simulink model "Flap"  (R2024b)
settings: Solver=ode45  StartTime=0  StopTime=400  FixedStep=0.1  MaxStep=0.1  EnableMultiTasking=on
values from neighbouring files (symbols this model uses):
  Ki = -2*pi/5*imag(1/H(1)')    [BranchAndBound.m]    (also in Optimization.m; RectangularOptimization.m; RoundingPI.m; wecSimInputFile.m = -100000)
  Kp = real(1/H(1)')    [BranchAndBound.m]    (also in Optimization.m; RectangularOptimization.m; RoundingPI.m; wecSimInputFile.m = 500000)
  params = struct    [BranchAndBound.m]    (also in Optimization.m; Parameters.m = struct(); RectangularOptimization.m; RoundingPI.m)
  PTO = 'Continuous PI'    [wecSimInputFile.m]
  valveTransferFunction = tf(4/valveSettlingTime,[1 4/valveSettlingTime])    [Parameters.m]
undefined symbols (not defined in the file or in its folder): body, constraint, geometry, hydroData, pressure, pto, ptoSim
libraries: WECSim_Lib_Body_Elements x2, WECSim_Lib_Constraints x1, WECSim_Lib_Frames x1, simulink x1, WECSim_Lib_PTOSim x1, WECSim_Lib_PTOs x1
(part 1 of 2)
settings Model: Creator=mlawson  LastModifiedBy=jackson
settings SolverCC: ZeroCrossControl=DisableAll  AlgebraicLoopSolver=LineSearch  AutoInsertRateTranBlk=on
settings DataIOCC: SaveFormat=Array  SaveOutput=off  SaveTime=off  ReturnWorkspaceOutputs=off
settings OptimizationCC: LifeSpan=inf  SimCompilerOptimization=on
settings DebuggingCC: MergeDetectMultiDrivingBlocksExec=none  SolverPrmCheckMsg=warning  UnconnectedInputMsg=warning  UnconnectedOutputMsg=warning  UnconnectedLineMsg=warning  AllowSymbolicDim=off  StateNameClashWarn=warning  SFUnexpectedBacktrackingDiag=warning  SFNoUnconditionalDefaultTransitionDiag=warning  SFExecutionAtInitializationDiag=none  ArithmeticOperatorsInVariantConditions=warning
settings HardwareCC: ProdBitPerPointer=32  ProdBitPerSizeT=32  ProdBitPerPtrDiffT=32  ProdLargestAtomicFloat=None  ProdIntDivRoundTo=Undefined  ProdEndianess=Unspecified  ProdWordSize=32  ProdHWDeviceType=32-bit Generic
settings ModelReferenceCC: EnableRefExpFcnMdlSchedulingChecks=on  PropagateSignalLabelsOutOfModel=off
settings SFSimCC: SimUseLocalCustomCode=off  CustomCodeUndefinedFunction=UseInterfaceOnly
settings RTWCC: RTWUseLocalCustomCode=off  GPUComputeCapability=3.5  DLArmComputeVersion=19.05
settings CodeAppCC: StateflowObjectComments=on
settings GRTTargetCC: TargetLangStandard=C89/C90 (ANSI)
settings ConfigComp: CovMetricSettings=dw  CovSaveCumulativeToWorkspaceVar=on  CovSaveSingleToWorkspaceVar=on  CovExternalEMLEnable=off  CovSFcnEnable=off
settings SimscapeCC: SimscapeNormalizeSystem=off
settings ConfigurationSet: Description=SimMechanics 2G
settings ExplorerConfigSet: InternalSimMechanicsExplorerSettings="<ExplorerConfiguration><canonicalview>default</canonicalview><TilePanel><TileInfo><Tiles Columns=\"1\" Count=\"1\" Rows=\"1\"><Column Left=\"2\" Weight=\"1\"/><Column Left=\"1335\"/><Row Top=\"2\" Weight=\"1\"/><Row Top=\"911\"/><Tile Height=\"1\" Width=\"1\" X=\"0\" Y=\"0\"/></Tiles></TileInfo><SceneInfo><SceneViewer><BGColor><R>0.60000002384185791</R><G>0.60000002384185791</G><B>0.60000002384185791</B></BGColor><Camera><Position><X>365.37645888990272</X><Y>-369.82486814446582</Y><Z>359.64809521743916</Z></Position><Center><X>-6.7351450971904585</X><Y>2.2867358426280204</Y><Z>-12.463508769654169</Z></Center><Up><X>-0.40824829046386307</X><Y>0.40824829046386307</Y><Z>0.81649658092772615</Z></Up><Left>-57.820127362122818</Left><Right>57.820127362122818</Right><Bottom>-38.308817187253304</Bottom><Top>38.308817187253304</Top></Camera></SceneViewer></SceneInfo></TilePanel></ExplorerConfiguration>"

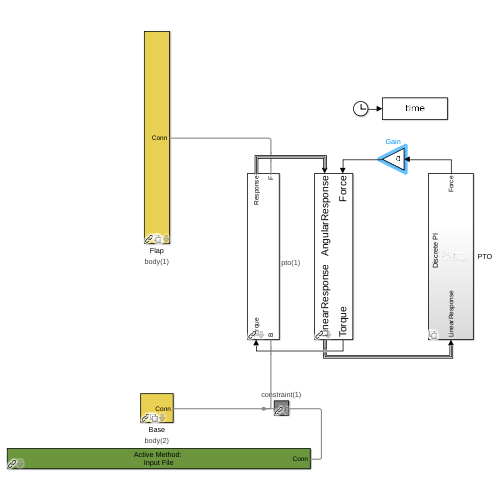
[thumbnail: Simulink's stored preview of the top-level diagram]
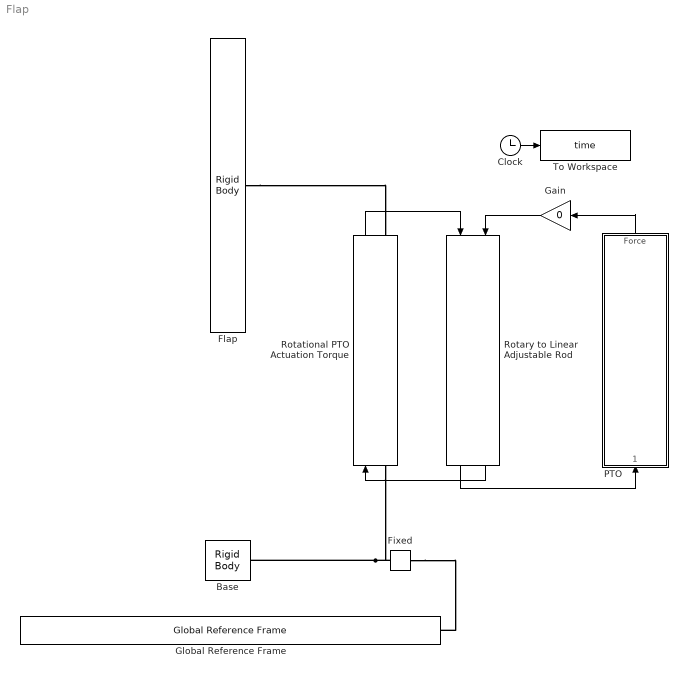
== system Flap ==
  Base : WECSim_Lib_Body_Elements/Rigid Body  body=body(2)  h5File=hydroData/*.h5  geometryFile=geometry/*.stl  mass=0  inertia=0 0 0  inertiaProducts=0 0 0  nonHydro=0  nonlinearHydro=0  centerGravity=0 0 0  centerBuoyancy=0 0 0  dof=6  volume=0  QTFs=0  displacement=0 0 0  axis=0 1 0  angle=0  option=0  cd=0 0 0  ca=0 0 0  area=0 0 0  VME=0  rgME=0 0 0  z=0 0 1
      settings: SourceProductName=WEC-Sim
  Clock : Clock
  Fixed : WECSim_Lib_Constraints/Fixed  constraint=constraint(1)  loc="0  0  0"  displacement=0 0 0  y=0 1 0  z=0 0 1  upperLimitSpecify=off  upperLimitBound=0  upperLimitTransitionRegionWidth=0  upperLimitStiffness=0  upperLimitDamping=0  lowerLimitSpecify=off  lowerLimitBound=0  lowerLimitTransitionRegionWidth=0  lowerLimitStiffness=0  lowerLimitDamping=0
      settings: AttributesFormatString=%<constraint>  SourceProductName=WEC-Sim
  Flap : WECSim_Lib_Body_Elements/Rigid Body  body=body(1)  h5File=hydroData/*.h5  geometryFile=geometry/*.stl  mass=0  inertia=0 0 0  inertiaProducts=0 0 0  nonHydro=0  nonlinearHydro=0  centerGravity=0 0 0  centerBuoyancy=0 0 0  dof=6  volume=0  QTFs=0  displacement=0 0 0  axis=0 1 0  angle=0  option=0  cd=0 0 0  ca=0 0 0  area=0 0 0  VME=0  rgME=0 0 0  z=0 0 1
      settings: SourceProductName=WEC-Sim
  Gain : Gain  Gain=0
  Global Reference Frame : WECSim_Lib_Frames/Global Reference Frame  waves=waves  simu=simu  InputMethod=Input File  InputFile=wecSimInputFile.m  mode=normal  explorer=off  solver=ode4  startTime=0  rampTime=100  endTime=400  dt=0.1  cicEndTime=60  stateSpace=0  WaveClass=regular  height=2.5  period=8  elevationFile=NOT DEFINED  spectrumFile=NOT DEFINED  direction=0  spread=1  spectrumType=NOT DEFINED  phaseSeed=0  option=EqualEnergy
      settings: SourceProductName=WEC-Sim
  PTO : Subsystem  Variant=on
  Rotary to Linear Adjustable Rod : WECSim_Lib_PTOSim/Motion Conversion/Rotary to Linear Adjustable Rod  ptoSim=ptoSim(1)  crank=crank_z  offset=0  rodInit=initalCylinderLength
  Rotational PTO Actuation Torque : WECSim_Lib_PTOs/Rotational PTO Actuation Torque  pto=pto(1)  loc="0  0  0"  stiffness=0  damping=0  equilibriumPosition=0  pretension=0  displacement=0 0 0  y=0 1 0  z=0 0 1  upperLimitSpecify=off  upperLimitBound=0  upperLimitTransitionRegionWidth=0  upperLimitStiffness=0  upperLimitDamping=0  lowerLimitSpecify=off  lowerLimitBound=0  lowerLimitTransitionRegionWidth=0  lowerLimitStiffness=0  lowerLimitDamping=0
      settings: AttributesFormatString=%<pto>
  To Workspace : ToWorkspace  VariableName=time  SampleTime=-1
  wires:
  Rotational PTO Actuation Torque/1 -> Rotary to Linear Adjustable Rod/1
  Rotary to Linear Adjustable Rod/2 -> Rotational PTO Actuation Torque/1
  Rotary to Linear Adjustable Rod/1 -> PTO/1(LinearResponse)
  PTO/1(Force) -> Gain/1
  Clock/1 -> To Workspace/1
  Gain/1 -> Rotary to Linear Adjustable Rod/2
  connections:
  Fixed/LConn1 -- Global Reference Frame/RConn1
  Fixed/RConn1 -- Base/RConn1 -- Rotational PTO Actuation Torque/LConn1
  Flap/RConn1 -- Rotational PTO Actuation Torque/RConn1

== system Flap/PTO ==
  note: 1) Add Subsystem or Model blocks as valid variant choices.
      | 2) You cannot connect blocks at this level. At simulation, connectivity is automatically
      | determined, based on the active variant and port name matching.
  LinearResponse : Inport
  Active Valving : Subsystem  VariantControl=strcmp(PTO, 'Active Valving')
  Continuous PI : Subsystem  VariantControl=strcmp(PTO, 'Continuous PI')
  Discrete PI : Subsystem  VariantControl=strcmp(PTO, 'Discrete PI')
  EHA : Subsystem  VariantControl=strcmp(PTO, 'EHA')
  HHEA : Subsystem  VariantControl=strcmp(PTO, 'HHEA')
  Passive Valving : Subsystem  VariantControl=strcmp(PTO, 'Passive Valving')
  Rectifying : Subsystem  VariantControl=strcmp(PTO, 'Rectifying')
  Force : Outport

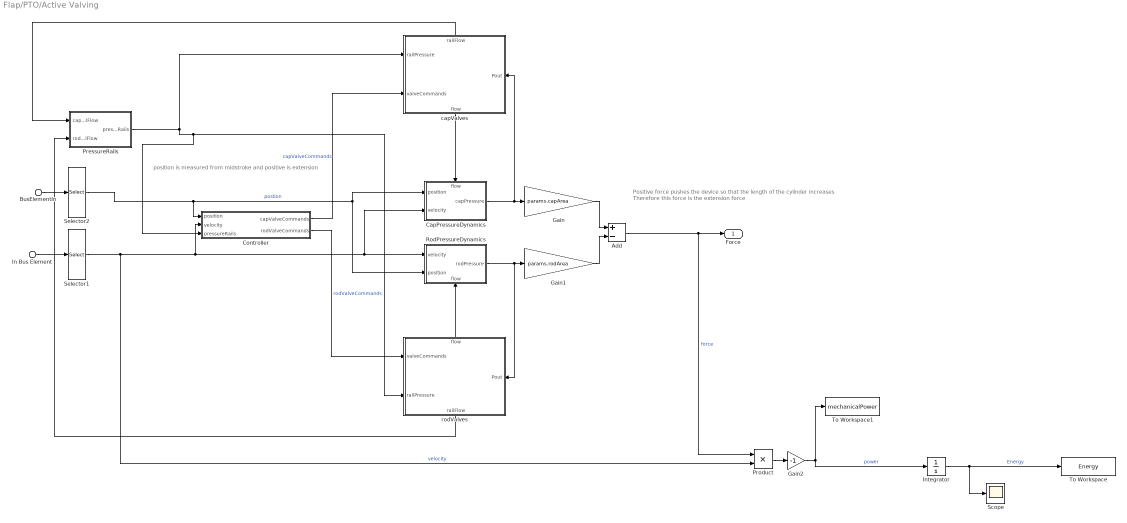
== system Flap/PTO/Active Valving ==
  note: position is measured from midstroke and positive is extension
  note: Positive force pushes the device so that the length of the cylinder increases
      | Therefore this force is the extension force
  In Bus Element : Inport  PortName=LinearResponse  Element=velocity
  BusElementIn : Inport  PortName=LinearResponse  Element=position
  Add : Sum  Inputs=+-
  CapPressureDynamics : Subsystem
      settings: PortSchema="{\"entries\":[{\"content\":{\"sides\":[{\"content\":{\"connectorIds\":[\"In1\",\"In2\"]},\"type\":\"ConnectorPlacement.EquallySpacedRectSide\",\"uuid\":\"0a444e4d-7364-44e5-8b72-8c210fabafa0\"},{\"content\":{\"connectorIds\":[\"Out1\"],\"side\":\"RIGHT\"},\"type\":\"ConnectorPlacement.EquallySpacedRectSide\",\"uuid\":\"a3669697-8e2e-4fce-83e7-11feb3c41a11\"},{\"content\":{\"connectorIds\":[\"In3\"],\"side\":\"TOP\"},\"type\":\"ConnectorPlacement.EquallySpacedRectSide\",\"uuid\":\"edbd7469-179d-4b36-ab80-dceaa86ef763\"},{\"content\":{\"side\":\"BOTTOM\"},\"type\":\"ConnectorPlacement.EquallySpacedRectSide\",\"uuid\":\"36ba3990-6628-4e3d-ab1a-10917dd4fa0b\"}]},\"type\":\"ConnectorPlacement.EquallySpacedConnector\",\"uuid\":\"68480e3c-12c2-4c1a-9580-60c15ea9a162\"}],\"packageUris\":[\"http://schema.mathworks.com/mf0/Connector/R2020b\"],\"version\":\"1.0\"}"
  Controller : Subsystem
  Gain : Gain  Gain=params.capArea
  Gain1 : Gain  Gain=params.rodArea
  Gain2 : Gain  Gain=-1
  Integrator : Integrator
  PressureRails : Subsystem
  Product : Product
  RodPressureDynamics : Subsystem
      settings: PortSchema="{\"entries\":[{\"content\":{\"sides\":[{\"content\":{\"connectorIds\":[\"In1\",\"In2\"]},\"type\":\"ConnectorPlacement.EquallySpacedRectSide\",\"uuid\":\"0a444e4d-7364-44e5-8b72-8c210fabafa0\"},{\"content\":{\"connectorIds\":[\"Out1\"],\"side\":\"RIGHT\"},\"type\":\"ConnectorPlacement.EquallySpacedRectSide\",\"uuid\":\"a3669697-8e2e-4fce-83e7-11feb3c41a11\"},{\"content\":{\"side\":\"TOP\"},\"type\":\"ConnectorPlacement.EquallySpacedRectSide\",\"uuid\":\"edbd7469-179d-4b36-ab80-dceaa86ef763\"},{\"content\":{\"connectorIds\":[\"In3\"],\"side\":\"BOTTOM\"},\"type\":\"ConnectorPlacement.EquallySpacedRectSide\",\"uuid\":\"0057cc85-602f-4ff7-8e06-c43254199496\"}]},\"type\":\"ConnectorPlacement.EquallySpacedConnector\",\"uuid\":\"68480e3c-12c2-4c1a-9580-60c15ea9a162\"}],\"packageUris\":[\"http://schema.mathworks.com/mf0/Connector/R2020b\"],\"version\":\"1.0\"}"
  Scope : Scope
  Selector1 : Selector  InputPortWidth=6  IndexOptions=Index vector (dialog)  Indices=3  OutputSizes=1
  Selector2 : Selector  InputPortWidth=6  IndexOptions=Index vector (dialog)  Indices=3  OutputSizes=1
  To Workspace : ToWorkspace  VariableName=Energy  SampleTime=-1
      settings: MaxDataPoints=1
  To Workspace1 : ToWorkspace  VariableName=mechanicalPower  SampleTime=-1
  capValves : Subsystem
      settings: PortSchema="{\"entries\":[{\"content\":{\"sides\":[{\"content\":{\"connectorIds\":[\"In1\",\"In2\"]},\"type\":\"ConnectorPlacement.EquallySpacedRectSide\",\"uuid\":\"d2e8cfa0-a0ae-49da-8fda-082dfd3b2d9f\"},{\"content\":{\"connectorIds\":[\"In3\"],\"side\":\"RIGHT\"},\"type\":\"ConnectorPlacement.EquallySpacedRectSide\",\"uuid\":\"7b83af61-76d6-4e35-9365-fafdba130762\"},{\"content\":{\"connectorIds\":[\"Out2\"],\"side\":\"TOP\"},\"type\":\"ConnectorPlacement.EquallySpacedRectSide\",\"uuid\":\"6880d985-ed9d-415d-a1a9-fc8aaf1ae9e0\"},{\"content\":{\"connectorIds\":[\"Out1\"],\"side\":\"BOTTOM\"},\"type\":\"ConnectorPlacement.EquallySpacedRectSide\",\"uuid\":\"f70b92c7-c6bf-4dbf-a331-364ba55ce8fb\"}]},\"type\":\"ConnectorPlacement.EquallySpacedConnector\",\"uuid\":\"7ffcaf2b-fb7f-4cb0-b739-43ebea45fc90\"}],\"packageUris\":[\"http://schema.mathworks.com/mf0/Connector/R2020b\"],\"version\":\"1.0\"}"
  rodValves : Subsystem
      settings: PortSchema="{\"entries\":[{\"content\":{\"sides\":[{\"content\":{\"connectorIds\":[\"In1\",\"In2\"]},\"type\":\"ConnectorPlacement.EquallySpacedRectSide\",\"uuid\":\"d2e8cfa0-a0ae-49da-8fda-082dfd3b2d9f\"},{\"content\":{\"connectorIds\":[\"In3\"],\"side\":\"RIGHT\"},\"type\":\"ConnectorPlacement.EquallySpacedRectSide\",\"uuid\":\"7b83af61-76d6-4e35-9365-fafdba130762\"},{\"content\":{\"connectorIds\":[\"Out2\"],\"side\":\"TOP\"},\"type\":\"ConnectorPlacement.EquallySpacedRectSide\",\"uuid\":\"6880d985-ed9d-415d-a1a9-fc8aaf1ae9e0\"},{\"content\":{\"connectorIds\":[\"Out1\"],\"side\":\"BOTTOM\"},\"type\":\"ConnectorPlacement.EquallySpacedRectSide\",\"uuid\":\"f70b92c7-c6bf-4dbf-a331-364ba55ce8fb\"}]},\"type\":\"ConnectorPlacement.EquallySpacedConnector\",\"uuid\":\"7ffcaf2b-fb7f-4cb0-b739-43ebea45fc90\"}],\"packageUris\":[\"http://schema.mathworks.com/mf0/Connector/R2020b\"],\"version\":\"1.0\"}"
  Force : Outport
  wires:
  rodValves/2(flow) -> RodPressureDynamics/3(flow)
  Controller/2(rodValveCommands) -> rodValves/1(valveCommands)  "rodValveCommands"
  Controller/1(capValveCommands) -> capValves/2(valveCommands)  "capValveCommands"
  capValves/1(flow) -> CapPressureDynamics/3(flow)
  RodPressureDynamics/1(rodPressure) -> rodValves/3(Pout), Gain1/1
  PressureRails/1(pressureRails) -> capValves/1(railPressure), Controller/3(pressureRails), rodValves/2(railPressure)
  Gain1/1 -> Add/2
  CapPressureDynamics/1(capPressure) -> capValves/3(Pout), Gain/1
  Gain/1 -> Add/1
  BusElementIn/1 -> Selector2/1
  In Bus Element/1 -> Selector1/1
  Selector2/1 -> Controller/1(position), RodPressureDynamics/2(position), CapPressureDynamics/1(position)  "postion"
  Selector1/1 -> Product/2, Controller/2(velocity), RodPressureDynamics/1(velocity), CapPressureDynamics/2(velocity)  "velocity"
  Integrator/1 -> To Workspace/1, Scope/1  "Energy"
  Add/1 -> Product/1, Force/1  "force"
  rodValves/1(railFlow) -> PressureRails/2(rodRailFlow)
  capValves/2(railFlow) -> PressureRails/1(capRailFlow)
  Gain2/1 -> Integrator/1, To Workspace1/1  "power"
  Product/1 -> Gain2/1

== system Flap/PTO/Continuous PI ==
  note: Positive force pushes the device so that the length of the cylinder increases
      | Therefore this force is the extension force
  In Bus Element : Inport  PortName=LinearResponse  Element=velocity
  BusElementIn : Inport  PortName=LinearResponse  Element=position
  Gain : Gain  Gain=-Ki
  Gain1 : Gain  Gain=-Kp
  Integrator : Integrator
  Product : Product
  Scope : Scope
  Scope1 : Scope  NumInputPorts=2
  Selector1 : Selector  InputPortWidth=6  IndexOptions=Index vector (dialog)  Indices=3  OutputSizes=1
  Selector2 : Selector  InputPortWidth=6  IndexOptions=Index vector (dialog)  Indices=3  OutputSizes=1
  Sum : Sum  Inputs=|++
  To Workspace : ToWorkspace  VariableName=Energy  SampleTime=-1
      settings: MaxDataPoints=1
  Force : Outport
  wires:
  BusElementIn/1 -> Selector2/1
  In Bus Element/1 -> Selector1/1
  Sum/1 -> Scope1/1, Product/1, Force/1  "force"
  Selector1/1 -> Scope1/2, Gain1/1, Product/2  "velocity"
  Gain/1 -> Sum/1
  Gain1/1 -> Sum/2
  Product/1 -> Integrator/1  "Power"
  Integrator/1 -> To Workspace/1, Scope/1  "Energy"
  Selector2/1 -> Gain/1  "length"

== system Flap/PTO/Discrete PI ==
  note: Positive force pushes the device so that the length of the cylinder increases
      | Therefore this force is the extension force
  In Bus Element : Inport  PortName=LinearResponse  Element=velocity
  BusElementIn : Inport  PortName=LinearResponse  Element=position
  Gain : Gain  Gain=-Ki
  Gain1 : Gain  Gain=-Kp
  Integrator : Integrator
  MATLAB Function : MATLAB Function  TreatAsAtomicUnit=on
  Product : Product
  Scope : Scope
  Scope1 : Scope  NumInputPorts=2
  Selector1 : Selector  InputPortWidth=6  IndexOptions=Index vector (dialog)  Indices=3  OutputSizes=1
  Selector2 : Selector  InputPortWidth=6  IndexOptions=Index vector (dialog)  Indices=3  OutputSizes=1
  Sum : Sum  Inputs=|++
  To Workspace : ToWorkspace  VariableName=Energy  SampleTime=-1
      settings: MaxDataPoints=1
  Force : Outport
  wires:
  Integrator/1 -> To Workspace/1, Scope/1  "Energy"
  Product/1 -> Integrator/1  "Power"
  Gain1/1 -> Sum/2
  Gain/1 -> Sum/1
  Selector1/1 -> Gain1/1, Product/2  "velocity"
  Selector2/1 -> Gain/1  "length"
  Sum/1 -> Scope1/1, MATLAB Function/1(forceContinuous)  "ContinuousForce"
  In Bus Element/1 -> Selector1/1
  BusElementIn/1 -> Selector2/1
  MATLAB Function/1(forceDiscrete) -> Force/1, Scope1/2, Product/1  "discreteForce"

== system Flap/PTO/EHA ==
  In Bus Element : Inport  PortName=LinearResponse  Element=velocity
  BusElementIn : Inport  PortName=LinearResponse  Element=position
  Controller : Subsystem
  Selector1 : Selector  InputPortWidth=6  IndexOptions=Index vector (dialog)  Indices=3  OutputSizes=1
  Selector2 : Selector  InputPortWidth=6  IndexOptions=Index vector (dialog)  Indices=3  OutputSizes=1
  Subsystem : Subsystem
  Force : Outport
  wires:
  Subsystem/2(capPressure) -> Controller/3(capPressure)
  In Bus Element/1 -> Selector1/1  "velcty"
  Subsystem/1(Force) -> Force/1
  BusElementIn/1 -> Selector2/1
  Selector2/1 -> Controller/1(position), Subsystem/1(position)  "postion"
  Selector1/1 -> Subsystem/3(velocity), Controller/2(velocity)  "velocity"
  Controller/1(displacementCommand) -> Subsystem/2(displacementCommand)
  Subsystem/3(rodPressure) -> Controller/4(rodPressure)

== system Flap/PTO/HHEA ==
  In Bus Element : Inport  PortName=LinearResponse  Element=velocity
  BusElementIn : Inport  PortName=LinearResponse  Element=position
  Controller : Subsystem
  Selector1 : Selector  InputPortWidth=6  IndexOptions=Index vector (dialog)  Indices=3  OutputSizes=1
  Selector2 : Selector  InputPortWidth=6  IndexOptions=Index vector (dialog)  Indices=3  OutputSizes=1
  Subsystem : Subsystem
  Force : Outport
  wires:
  Controller/3("dP_command ") -> Subsystem/4("rodPressureCommand ")
  Subsystem/3(capPressure) -> Controller/4(capPressure)
  Controller/1(capValveCommands) -> Subsystem/2(capValveCommands)  "capValveCommands"
  Subsystem/4(rodValvePressure) -> Controller/5(rodValvePressure)
  In Bus Element/1 -> Selector1/1  "velcty"
  Subsystem/1(Force) -> Force/1
  Controller/2(rodValveCommands) -> Subsystem/3(rodValveCommands)  "rodValveCommands"
  BusElementIn/1 -> Selector2/1
  Subsystem/2(railPressure) -> Controller/3(pressureRails)
  Selector2/1 -> Controller/1(position), Subsystem/1(position)  "postion"
  Selector1/1 -> Subsystem/6(velocity), Controller/2(velocity)  "velocity"
  Controller/4(speedCommand) -> Subsystem/5(speedCommand)
  Subsystem/5(rodPressure) -> Controller/6(rodPressure)

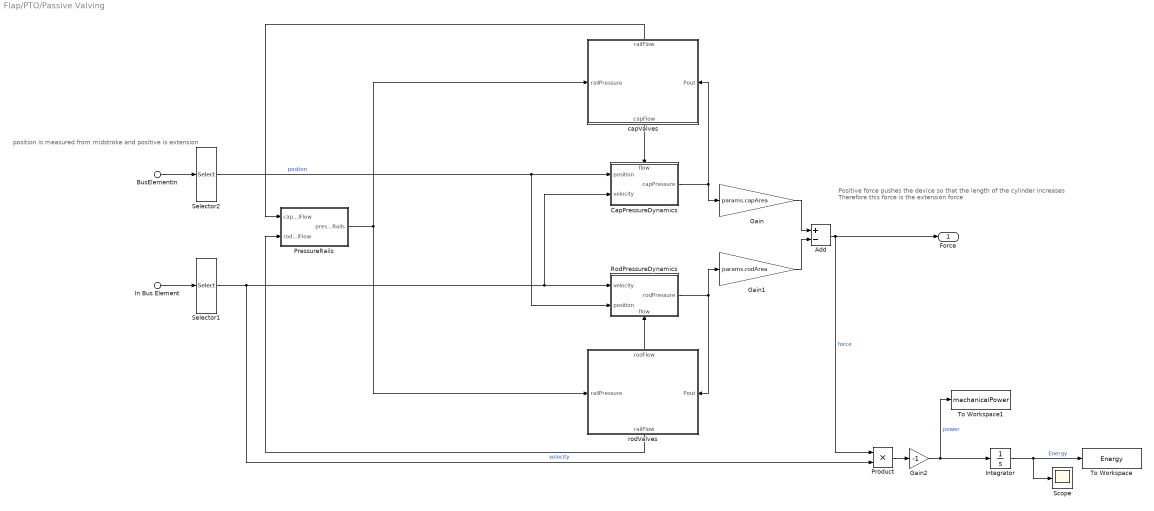
== system Flap/PTO/Passive Valving ==
  note: Positive force pushes the device so that the length of the cylinder increases
      | Therefore this force is the extension force
  note: position is measured from midstroke and positive is extension
  In Bus Element : Inport  PortName=LinearResponse  Element=velocity
  BusElementIn : Inport  PortName=LinearResponse  Element=position
  Add : Sum  Inputs=+-
  CapPressureDynamics : Subsystem
      settings: PortSchema="{\"entries\":[{\"content\":{\"sides\":[{\"content\":{\"connectorIds\":[\"In1\",\"In2\"]},\"type\":\"ConnectorPlacement.EquallySpacedRectSide\",\"uuid\":\"0a444e4d-7364-44e5-8b72-8c210fabafa0\"},{\"content\":{\"connectorIds\":[\"Out1\"],\"side\":\"RIGHT\"},\"type\":\"ConnectorPlacement.EquallySpacedRectSide\",\"uuid\":\"a3669697-8e2e-4fce-83e7-11feb3c41a11\"},{\"content\":{\"connectorIds\":[\"In3\"],\"side\":\"TOP\"},\"type\":\"ConnectorPlacement.EquallySpacedRectSide\",\"uuid\":\"edbd7469-179d-4b36-ab80-dceaa86ef763\"},{\"content\":{\"side\":\"BOTTOM\"},\"type\":\"ConnectorPlacement.EquallySpacedRectSide\",\"uuid\":\"36ba3990-6628-4e3d-ab1a-10917dd4fa0b\"}]},\"type\":\"ConnectorPlacement.EquallySpacedConnector\",\"uuid\":\"68480e3c-12c2-4c1a-9580-60c15ea9a162\"}],\"packageUris\":[\"http://schema.mathworks.com/mf0/Connector/R2020b\"],\"version\":\"1.0\"}"
  Gain : Gain  Gain=params.capArea
  Gain1 : Gain  Gain=params.rodArea
  Gain2 : Gain  Gain=-1
  Integrator : Integrator
  PressureRails : Subsystem
  Product : Product
  RodPressureDynamics : Subsystem
      settings: PortSchema="{\"entries\":[{\"content\":{\"sides\":[{\"content\":{\"connectorIds\":[\"In1\",\"In2\"]},\"type\":\"ConnectorPlacement.EquallySpacedRectSide\",\"uuid\":\"0a444e4d-7364-44e5-8b72-8c210fabafa0\"},{\"content\":{\"connectorIds\":[\"Out1\"],\"side\":\"RIGHT\"},\"type\":\"ConnectorPlacement.EquallySpacedRectSide\",\"uuid\":\"a3669697-8e2e-4fce-83e7-11feb3c41a11\"},{\"content\":{\"side\":\"TOP\"},\"type\":\"ConnectorPlacement.EquallySpacedRectSide\",\"uuid\":\"edbd7469-179d-4b36-ab80-dceaa86ef763\"},{\"content\":{\"connectorIds\":[\"In3\"],\"side\":\"BOTTOM\"},\"type\":\"ConnectorPlacement.EquallySpacedRectSide\",\"uuid\":\"0057cc85-602f-4ff7-8e06-c43254199496\"}]},\"type\":\"ConnectorPlacement.EquallySpacedConnector\",\"uuid\":\"68480e3c-12c2-4c1a-9580-60c15ea9a162\"}],\"packageUris\":[\"http://schema.mathworks.com/mf0/Connector/R2020b\"],\"version\":\"1.0\"}"
  Scope : Scope
  Selector1 : Selector  InputPortWidth=6  IndexOptions=Index vector (dialog)  Indices=3  OutputSizes=1
  Selector2 : Selector  InputPortWidth=6  IndexOptions=Index vector (dialog)  Indices=3  OutputSizes=1
  To Workspace : ToWorkspace  VariableName=Energy  SampleTime=-1
      settings: MaxDataPoints=1
  To Workspace1 : ToWorkspace  VariableName=mechanicalPower  SampleTime=-1
  capValves : Subsystem
      settings: PortSchema="{\"entries\":[{\"content\":{\"sides\":[{\"content\":{\"connectorIds\":[\"In1\"]},\"type\":\"ConnectorPlacement.EquallySpacedRectSide\",\"uuid\":\"d2e8cfa0-a0ae-49da-8fda-082dfd3b2d9f\"},{\"content\":{\"connectorIds\":[\"In2\"],\"side\":\"RIGHT\"},\"type\":\"ConnectorPlacement.EquallySpacedRectSide\",\"uuid\":\"7b83af61-76d6-4e35-9365-fafdba130762\"},{\"content\":{\"connectorIds\":[\"Out2\"],\"side\":\"TOP\"},\"type\":\"ConnectorPlacement.EquallySpacedRectSide\",\"uuid\":\"6880d985-ed9d-415d-a1a9-fc8aaf1ae9e0\"},{\"content\":{\"connectorIds\":[\"Out1\"],\"side\":\"BOTTOM\"},\"type\":\"ConnectorPlacement.EquallySpacedRectSide\",\"uuid\":\"f70b92c7-c6bf-4dbf-a331-364ba55ce8fb\"}]},\"type\":\"ConnectorPlacement.EquallySpacedConnector\",\"uuid\":\"7ffcaf2b-fb7f-4cb0-b739-43ebea45fc90\"}],\"packageUris\":[\"http://schema.mathworks.com/mf0/Connector/R2020b\"],\"version\":\"1.0\"}"
  rodValves : Subsystem
      settings: PortSchema="{\"entries\":[{\"content\":{\"sides\":[{\"content\":{\"connectorIds\":[\"In1\"]},\"type\":\"ConnectorPlacement.EquallySpacedRectSide\",\"uuid\":\"d2e8cfa0-a0ae-49da-8fda-082dfd3b2d9f\"},{\"content\":{\"connectorIds\":[\"In2\"],\"side\":\"RIGHT\"},\"type\":\"ConnectorPlacement.EquallySpacedRectSide\",\"uuid\":\"7b83af61-76d6-4e35-9365-fafdba130762\"},{\"content\":{\"connectorIds\":[\"Out2\"],\"side\":\"TOP\"},\"type\":\"ConnectorPlacement.EquallySpacedRectSide\",\"uuid\":\"6880d985-ed9d-415d-a1a9-fc8aaf1ae9e0\"},{\"content\":{\"connectorIds\":[\"Out1\"],\"side\":\"BOTTOM\"},\"type\":\"ConnectorPlacement.EquallySpacedRectSide\",\"uuid\":\"f70b92c7-c6bf-4dbf-a331-364ba55ce8fb\"}]},\"type\":\"ConnectorPlacement.EquallySpacedConnector\",\"uuid\":\"7ffcaf2b-fb7f-4cb0-b739-43ebea45fc90\"}],\"packageUris\":[\"http://schema.mathworks.com/mf0/Connector/R2020b\"],\"version\":\"1.0\"}"
  Force : Outport
  wires:
  Add/1 -> Force/1, Product/1  "force"
  Product/1 -> Gain2/1
  Integrator/1 -> Scope/1, To Workspace/1  "Energy"
  Selector1/1 -> CapPressureDynamics/2(velocity), RodPressureDynamics/1(velocity), Product/2  "velocity"
  Selector2/1 -> RodPressureDynamics/2(position), CapPressureDynamics/1(position)  "postion"
  In Bus Element/1 -> Selector1/1
  BusElementIn/1 -> Selector2/1
  Gain/1 -> Add/1
  CapPressureDynamics/1(capPressure) -> Gain/1, capValves/2(Pout)
  Gain1/1 -> Add/2
  RodPressureDynamics/1(rodPressure) -> Gain1/1, rodValves/2(Pout)
  capValves/1(capFlow) -> CapPressureDynamics/3(flow)
  rodValves/2(rodFlow) -> RodPressureDynamics/3(flow)
  PressureRails/1(pressureRails) -> capValves/1(railPressure), rodValves/1(railPressure)
  capValves/2(railFlow) -> PressureRails/1(capRailFlow)
  rodValves/1(railFlow) -> PressureRails/2(rodRailFlow)
  Gain2/1 -> Integrator/1, To Workspace1/1  "power"

== system Flap/PTO/Rectifying ==
  note: Positive force pushes the device so that the length of the cylinder increases
      | Therefore this force is the extension force
  In Bus Element : Inport  PortName=LinearResponse  Element=velocity
  BusElementIn : Inport  PortName=LinearResponse  Element=position
  Constant : Constant  Value=pressure
  Integrator : Integrator
  MATLAB Function : MATLAB Function  TreatAsAtomicUnit=on
  Product : Product
  Scope : Scope
  Scope1 : Scope  NumInputPorts=2
  Selector1 : Selector  InputPortWidth=6  IndexOptions=Index vector (dialog)  Indices=3  OutputSizes=1
  Selector2 : Selector  InputPortWidth=6  IndexOptions=Index vector (dialog)  Indices=3  OutputSizes=1
  Terminator : Terminator
  To Workspace : ToWorkspace  VariableName=Energy  SampleTime=-1
      settings: MaxDataPoints=1
  Force : Outport
  wires:
  Integrator/1 -> To Workspace/1, Scope/1  "Energy"
  Product/1 -> Integrator/1  "Power"
  Selector1/1 -> MATLAB Function/1(velocity), Scope1/1, Product/2  "velocity"
  MATLAB Function/1(forceRectified) -> Scope1/2, Product/1, Force/1
  Constant/1 -> MATLAB Function/2(pressure)
  In Bus Element/1 -> Selector1/1
  BusElementIn/1 -> Selector2/1
  Selector2/1 -> Terminator/1  "position"

== system Flap/PTO/Active Valving/CapPressureDynamics ==
  position : Inport
  velocity : Inport  Port=2
  flow : Inport  Port=3
  Integrator : Integrator  LimitOutput=on  UpperSaturationLimit=40e6  LowerSaturationLimit=0
  MATLAB Function : MATLAB Function  TreatAsAtomicUnit=on
  capPressure : Outport
  wires:
  MATLAB Function/1(pressure_dot) -> Integrator/1
  Integrator/1 -> capPressure/1  "capPressure"
  flow/1 -> MATLAB Function/3(flow)
  velocity/1 -> MATLAB Function/2(velocity)
  position/1 -> MATLAB Function/1(position)

== system Flap/PTO/Active Valving/Controller ==
  position : Inport
  velocity : Inport  Port=2
  pressureRails : Inport  Port=3
  Gain : Gain  Gain=-params.Ki
  Gain1 : Gain  Gain=-params.Kp
  MATLAB Function : MATLAB Function  TreatAsAtomicUnit=on
  Scope1 : Scope  NumInputPorts=2
  Sum : Sum  Inputs=|++
  Terminator : Terminator
  Terminator1 : Terminator
  Zero-Order Hold : ZeroOrderHold  SampleTime=.2
  Zero-Order Hold1 : ZeroOrderHold  SampleTime=.2
  capValveCommands : Outport
  rodValveCommands : Outport  Port=2
  wires:
  velocity/1 -> Gain1/1  "velocity"
  Gain1/1 -> Sum/2
  Gain/1 -> Sum/1
  Sum/1 -> Scope1/1, MATLAB Function/1(forceContinuous)  "forceContinuous"
  MATLAB Function/3(forceDiscrete) -> Scope1/2  "forceDiscrete"
  position/1 -> Gain/1  "position"
  MATLAB Function/1(capValveCommands) -> Zero-Order Hold/1
  pressureRails/1 -> MATLAB Function/2(pressureRails)
  MATLAB Function/4(capPressureCommand) -> Terminator/1  "capPressureCommand"
  MATLAB Function/5(rodPressureCommand) -> Terminator1/1  "rodPressureCommand"
  Zero-Order Hold/1 -> capValveCommands/1
  MATLAB Function/2(rodValveCommands) -> Zero-Order Hold1/1
  Zero-Order Hold1/1 -> rodValveCommands/1

== system Flap/PTO/Active Valving/PressureRails ==
  note: flow into the rails
  capRailFlow : Inport
  rodRailFlow : Inport  Port=2
  Constant : Constant  Value=35e6
  Constant3 : Constant  Value=17.5e6
  Constant4 : Constant  Value=0
  Mux : Mux  Inputs=3
  Product : Product
  Sum : Sum  Inputs=|++
  Sum of Elements : Sum  Inputs=+
  To Workspace : ToWorkspace  VariableName=railPower  SampleTime=-1
  pressureRails : Outport
  wires:
  Sum/1 -> Product/1
  Product/1 -> Sum of Elements/1
  Sum of Elements/1 -> To Workspace/1
  rodRailFlow/1 -> Sum/2
  capRailFlow/1 -> Sum/1
  Constant3/1 -> Mux/2
  Constant4/1 -> Mux/1
  Constant/1 -> Mux/3
  Mux/1 -> Product/2, pressureRails/1

== system Flap/PTO/Active Valving/RodPressureDynamics ==
  velocity : Inport
  position : Inport  Port=2
  flow : Inport  Port=3
  Integrator : Integrator  LimitOutput=on  UpperSaturationLimit=40e6  LowerSaturationLimit=0
  MATLAB Function : MATLAB Function  TreatAsAtomicUnit=on
  rodPressure : Outport
  wires:
  position/1 -> MATLAB Function/1(position)
  velocity/1 -> MATLAB Function/2(velocity)
  flow/1 -> MATLAB Function/3(flow)
  Integrator/1 -> rodPressure/1  "rodPressure"
  MATLAB Function/1(pressure_dot) -> Integrator/1

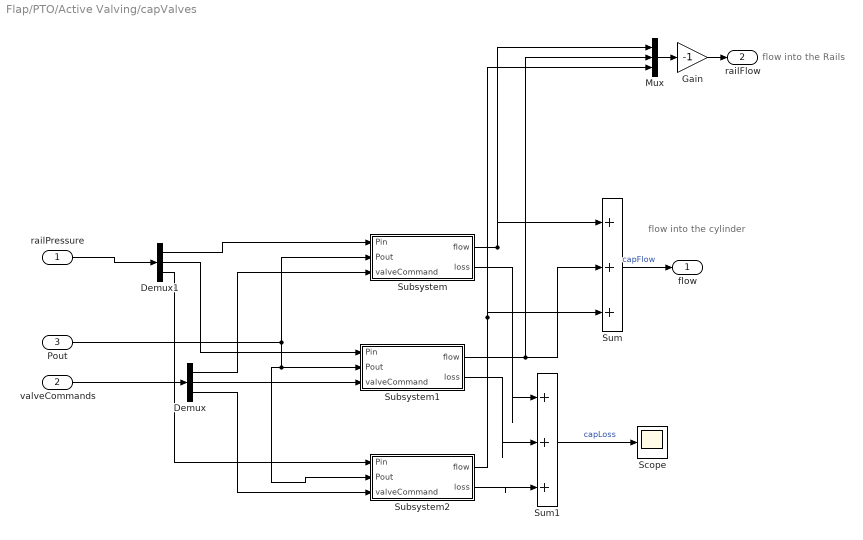
== system Flap/PTO/Active Valving/capValves ==
  note: flow into the cylinder
  note: flow into the Rails
  railPressure : Inport
  valveCommands : Inport  Port=2
  Pout : Inport  Port=3
  Demux : Demux  Outputs=3
  Demux1 : Demux  Outputs=3
  Gain : Gain  Gain=-1
  Mux : Mux  Inputs=3
  Scope : Scope
  Subsystem : Subsystem
  Subsystem1 : Subsystem
  Subsystem2 : Subsystem
  Sum : Sum  Inputs=|+++
  Sum1 : Sum  Inputs=|+++
  flow : Outport
  railFlow : Outport  Port=2
  wires:
  Pout/1 -> Subsystem/2(Pout), Subsystem2/2(Pout), Subsystem1/2(Pout)
  valveCommands/1 -> Demux/1
  Demux/1 -> Subsystem/3(valveCommand)
  Demux/2 -> Subsystem1/3(valveCommand)
  Demux/3 -> Subsystem2/3(valveCommand)
  Sum/1 -> flow/1  "capFlow"
  Subsystem/2(loss) -> Sum1/1
  Subsystem1/2(loss) -> Sum1/2
  Subsystem2/2(loss) -> Sum1/3
  Sum1/1 -> Scope/1  "capLoss"
  railPressure/1 -> Demux1/1
  Demux1/1 -> Subsystem/1(Pin)
  Demux1/2 -> Subsystem1/1(Pin)
  Demux1/3 -> Subsystem2/1(Pin)
  Mux/1 -> Gain/1
  Subsystem1/1(flow) -> Mux/2, Sum/2
  Gain/1 -> railFlow/1
  Subsystem/1(flow) -> Mux/1, Sum/1
  Subsystem2/1(flow) -> Mux/3, Sum/3

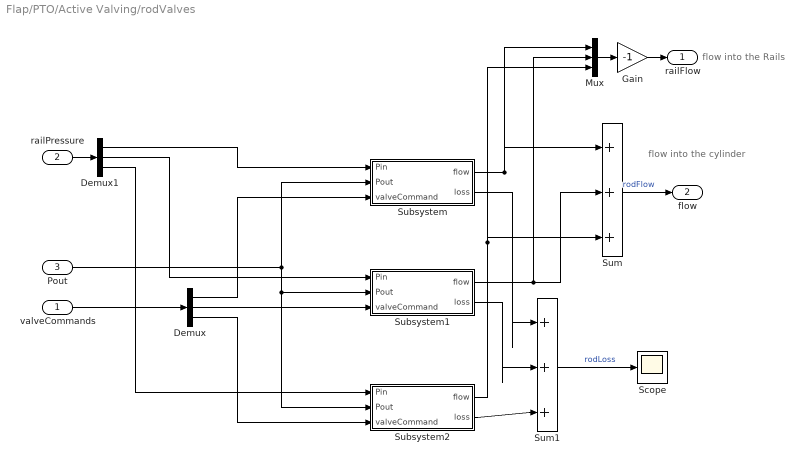
== system Flap/PTO/Active Valving/rodValves ==
  note: flow into the cylinder
  note: flow into the Rails
  valveCommands : Inport
  railPressure : Inport  Port=2
  Pout : Inport  Port=3
  Demux : Demux  Outputs=3
  Demux1 : Demux  Outputs=3
  Gain : Gain  Gain=-1
  Mux : Mux  Inputs=3
  Scope : Scope
  Subsystem : Subsystem
  Subsystem1 : Subsystem
  Subsystem2 : Subsystem
  Sum : Sum  Inputs=|+++
  Sum1 : Sum  Inputs=|+++
  railFlow : Outport
  flow : Outport  Port=2
  wires:
  Pout/1 -> Subsystem/2(Pout), Subsystem2/2(Pout), Subsystem1/2(Pout)
  valveCommands/1 -> Demux/1
  Demux/1 -> Subsystem/3(valveCommand)
  Demux1/2 -> Subsystem1/1(Pin)
  Demux1/3 -> Subsystem2/1(Pin)
  Demux/2 -> Subsystem1/3(valveCommand)
  Demux/3 -> Subsystem2/3(valveCommand)
  Subsystem2/1(flow) -> Mux/3, Sum/3
  Sum/1 -> flow/1  "rodFlow"
  Subsystem/2(loss) -> Sum1/1
  Subsystem1/2(loss) -> Sum1/2
  Subsystem2/2(loss) -> Sum1/3
  Sum1/1 -> Scope/1  "rodLoss"
  railPressure/1 -> Demux1/1
  Demux1/1 -> Subsystem/1(Pin)
  Gain/1 -> railFlow/1
  Subsystem1/1(flow) -> Mux/2, Sum/2
  Mux/1 -> Gain/1
  Subsystem/1(flow) -> Mux/1, Sum/1

== system Flap/PTO/EHA/Controller ==
  note: positive displacement sends flow to the rod side, decreasing the PTO force
  position : Inport
  velocity : Inport  Port=2
  capPressure : Inport  Port=3
  rodPressure : Inport  Port=4
  Gain : Gain  Gain=-params.Ki
  Gain1 : Gain  Gain=-params.Kp
  Gain2 : Gain  Gain=params.rodArea
  Gain3 : Gain  Gain=params.rodArea
  Saturation : Saturate  UpperLimit=1  LowerLimit=-1
  Sum : Sum  Inputs=|++
  Sum1 : Sum  Inputs=|+-
  Sum2 : Sum  Inputs=|+-
  Transfer Fcn : TransferFcn  Numerator=[1e-6 1e-6]  Denominator=[1 0]
  displacementCommand : Outport
  wires:
  velocity/1 -> Gain1/1  "velocity"
  Gain1/1 -> Sum/2
  Gain/1 -> Sum/1
  Sum/1 -> Sum2/2  "forceDesired"
  position/1 -> Gain/1  "position"
  capPressure/1 -> Gain2/1
  Transfer Fcn/1 -> Saturation/1
  rodPressure/1 -> Gain3/1
  Saturation/1 -> displacementCommand/1  "displacementCommand"
  Gain2/1 -> Sum1/1
  Gain3/1 -> Sum1/2
  Sum1/1 -> Sum2/1  "forceActual"
  Sum2/1 -> Transfer Fcn/1

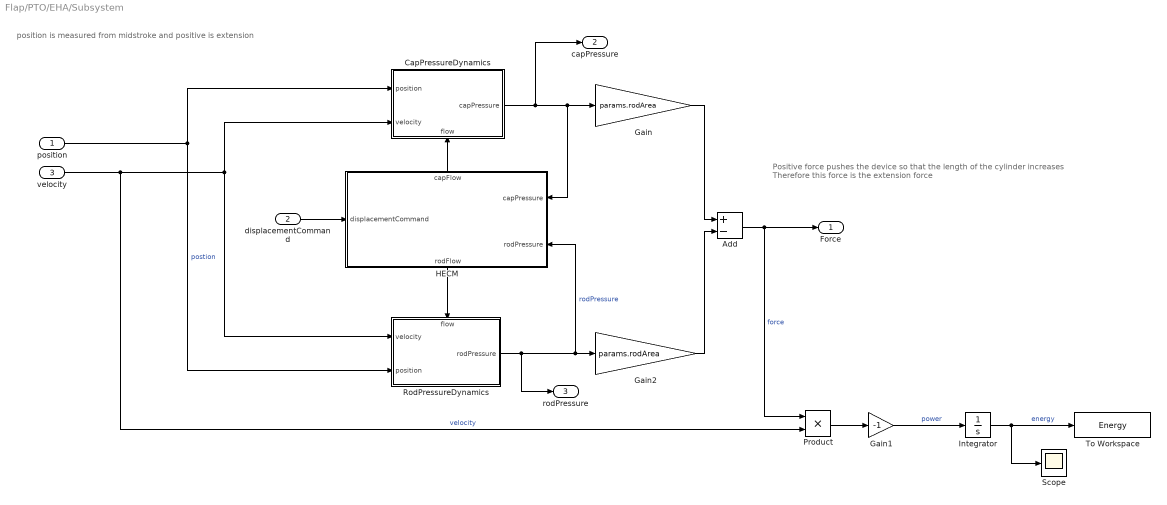
== system Flap/PTO/EHA/Subsystem ==
  note: position is measured from midstroke and positive is extension
  note: Positive force pushes the device so that the length of the cylinder increases
      | Therefore this force is the extension force
  position : Inport
  displacementCommand : Inport  Port=2
  velocity : Inport  Port=3
  Add : Sum  Inputs=+-
  CapPressureDynamics : Subsystem
      settings: PortSchema="{\"entries\":[{\"content\":{\"sides\":[{\"content\":{\"connectorIds\":[\"In1\",\"In2\"]},\"type\":\"ConnectorPlacement.EquallySpacedRectSide\",\"uuid\":\"0a444e4d-7364-44e5-8b72-8c210fabafa0\"},{\"content\":{\"connectorIds\":[\"Out1\"],\"side\":\"RIGHT\"},\"type\":\"ConnectorPlacement.EquallySpacedRectSide\",\"uuid\":\"a3669697-8e2e-4fce-83e7-11feb3c41a11\"},{\"content\":{\"side\":\"TOP\"},\"type\":\"ConnectorPlacement.EquallySpacedRectSide\",\"uuid\":\"edbd7469-179d-4b36-ab80-dceaa86ef763\"},{\"content\":{\"connectorIds\":[\"In3\"],\"side\":\"BOTTOM\"},\"type\":\"ConnectorPlacement.EquallySpacedRectSide\",\"uuid\":\"36ba3990-6628-4e3d-ab1a-10917dd4fa0b\"}]},\"type\":\"ConnectorPlacement.EquallySpacedConnector\",\"uuid\":\"68480e3c-12c2-4c1a-9580-60c15ea9a162\"}],\"packageUris\":[\"http://schema.mathworks.com/mf0/Connector/R2020b\"],\"version\":\"1.0\"}"
  Gain : Gain  Gain=params.rodArea
  Gain1 : Gain  Gain=-1
  Gain2 : Gain  Gain=params.rodArea
  HECM : Subsystem
      settings: PortSchema="{\"entries\":[{\"content\":{\"sides\":[{\"content\":{\"connectorIds\":[\"Out2\"]},\"type\":\"ConnectorPlacement.EquallySpacedRectSide\",\"uuid\":\"fa7e009b-3a28-4dd3-907b-76d8fd1f2fc5\"},{\"content\":{\"connectorIds\":[\"Out1\"],\"side\":\"RIGHT\"},\"type\":\"ConnectorPlacement.EquallySpacedRectSide\",\"uuid\":\"b4b71eb1-dc67-4897-9f20-563cedc71b8c\"},{\"content\":{\"connectorIds\":[\"In1\"],\"side\":\"TOP\"},\"type\":\"ConnectorPlacement.EquallySpacedRectSide\",\"uuid\":\"a67ddf4c-e1a7-4a41-beba-4c9482bc4896\"},{\"content\":{\"connectorIds\":[\"In2\",\"In3\"],\"side\":\"BOTTOM\"},\"type\":\"ConnectorPlacement.EquallySpacedRectSide\",\"uuid\":\"d70e9d30-0c3d-4fe1-994c-11171af7a54f\"}]},\"type\":\"ConnectorPlacement.EquallySpacedConnector\",\"uuid\":\"d5f93414-5adb-4b46-aa3e-a0fd5f50c915\"}],\"packageUris\":[\"http://schema.mathworks.com/mf0/Connector/R2020b\"],\"version\":\"1.0\"}"
  Integrator : Integrator
  Product : Product
  RodPressureDynamics : Subsystem
      settings: PortSchema="{\"entries\":[{\"content\":{\"sides\":[{\"content\":{\"connectorIds\":[\"In1\",\"In2\"]},\"type\":\"ConnectorPlacement.EquallySpacedRectSide\",\"uuid\":\"0a444e4d-7364-44e5-8b72-8c210fabafa0\"},{\"content\":{\"connectorIds\":[\"Out1\"],\"side\":\"RIGHT\"},\"type\":\"ConnectorPlacement.EquallySpacedRectSide\",\"uuid\":\"a3669697-8e2e-4fce-83e7-11feb3c41a11\"},{\"content\":{\"connectorIds\":[\"In3\"],\"side\":\"TOP\"},\"type\":\"ConnectorPlacement.EquallySpacedRectSide\",\"uuid\":\"edbd7469-179d-4b36-ab80-dceaa86ef763\"},{\"content\":{\"side\":\"BOTTOM\"},\"type\":\"ConnectorPlacement.EquallySpacedRectSide\",\"uuid\":\"0057cc85-602f-4ff7-8e06-c43254199496\"}]},\"type\":\"ConnectorPlacement.EquallySpacedConnector\",\"uuid\":\"68480e3c-12c2-4c1a-9580-60c15ea9a162\"}],\"packageUris\":[\"http://schema.mathworks.com/mf0/Connector/R2020b\"],\"version\":\"1.0\"}"
  Scope : Scope
  To Workspace : ToWorkspace  VariableName=Energy  SampleTime=-1
      settings: MaxDataPoints=1
  Force : Outport
  capPressure : Outport  Port=2
  rodPressure : Outport  Port=3
  wires:
  Gain/1 -> Add/1
  RodPressureDynamics/1(rodPressure) -> rodPressure/1, Gain2/1, HECM/2(rodPressure)  "rodPressure"
  HECM/1(capFlow) -> CapPressureDynamics/3(flow)
  position/1 -> CapPressureDynamics/1(position), RodPressureDynamics/2(position)  "postion"
  Integrator/1 -> To Workspace/1, Scope/1  "energy"
  velocity/1 -> Product/2, RodPressureDynamics/1(velocity), CapPressureDynamics/2(velocity)  "velocity"
  CapPressureDynamics/1(capPressure) -> capPressure/1, Gain/1, HECM/3(capPressure)
  Product/1 -> Gain1/1
  Add/1 -> Force/1, Product/1  "force"
  displacementCommand/1 -> HECM/1(displacementCommand)
  Gain2/1 -> Add/2
  HECM/2(rodFlow) -> RodPressureDynamics/3(flow)
  Gain1/1 -> Integrator/1  "power"

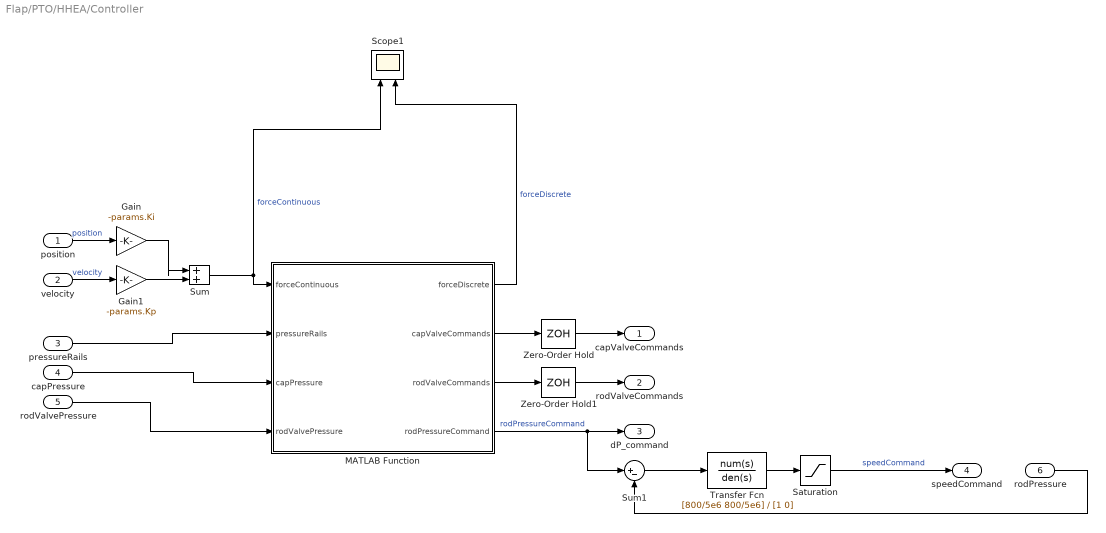
== system Flap/PTO/HHEA/Controller ==
  position : Inport
  velocity : Inport  Port=2
  pressureRails : Inport  Port=3
  capPressure : Inport  Port=4
  rodValvePressure : Inport  Port=5
  rodPressure : Inport  Port=6
  Gain : Gain  Gain=-params.Ki
  Gain1 : Gain  Gain=-params.Kp
  MATLAB Function : MATLAB Function  TreatAsAtomicUnit=on
  Saturation : Saturate  UpperLimit=1000  LowerLimit=-1000
  Scope1 : Scope  NumInputPorts=2
  Sum : Sum  Inputs=|++
  Sum1 : Sum  Inputs=|+-
  Transfer Fcn : TransferFcn  Numerator=[800/5e6 800/5e6]  Denominator=[1 0]
  Zero-Order Hold : ZeroOrderHold  SampleTime=.2
  Zero-Order Hold1 : ZeroOrderHold  SampleTime=.2
  capValveCommands : Outport
  rodValveCommands : Outport  Port=2
  "dP_command " : Outport  Port=3
  speedCommand : Outport  Port=4
  wires:
  velocity/1 -> Gain1/1  "velocity"
  Gain1/1 -> Sum/2
  Gain/1 -> Sum/1
  Sum/1 -> Scope1/1, MATLAB Function/1(forceContinuous)  "forceContinuous"
  MATLAB Function/1(forceDiscrete) -> Scope1/2  "forceDiscrete"
  position/1 -> Gain/1  "position"
  MATLAB Function/2(capValveCommands) -> Zero-Order Hold/1
  MATLAB Function/3(rodValveCommands) -> Zero-Order Hold1/1
  pressureRails/1 -> MATLAB Function/2(pressureRails)
  MATLAB Function/4(rodPressureCommand) -> "dP_command "/1, Sum1/1  "rodPressureCommand"
  capPressure/1 -> MATLAB Function/3(capPressure)
  rodValvePressure/1 -> MATLAB Function/4(rodValvePressure)
  Zero-Order Hold/1 -> capValveCommands/1
  Zero-Order Hold1/1 -> rodValveCommands/1
  Transfer Fcn/1 -> Saturation/1
  rodPressure/1 -> Sum1/2
  Sum1/1 -> Transfer Fcn/1
  Saturation/1 -> speedCommand/1  "speedCommand"

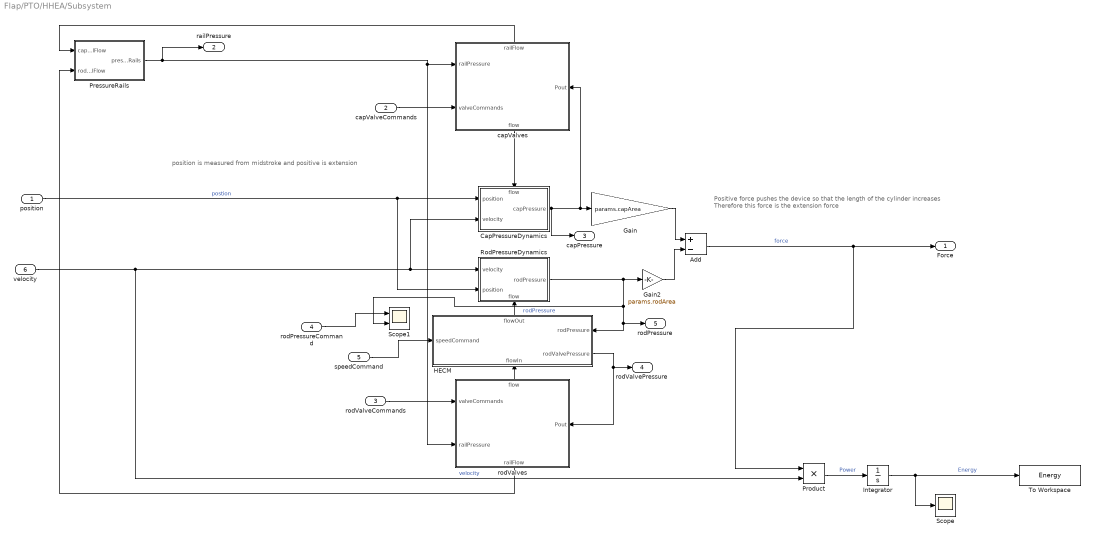
== system Flap/PTO/HHEA/Subsystem ==
  note: position is measured from midstroke and positive is extension
  note: Positive force pushes the device so that the length of the cylinder increases
      | Therefore this force is the extension force
  position : Inport
  capValveCommands : Inport  Port=2
  rodValveCommands : Inport  Port=3
  "rodPressureCommand " : Inport  Port=4
  speedCommand : Inport  Port=5
  velocity : Inport  Port=6
  Add : Sum  Inputs=+-
  CapPressureDynamics : Subsystem
      settings: PortSchema="{\"entries\":[{\"content\":{\"sides\":[{\"content\":{\"connectorIds\":[\"In1\",\"In2\"]},\"type\":\"ConnectorPlacement.EquallySpacedRectSide\",\"uuid\":\"0a444e4d-7364-44e5-8b72-8c210fabafa0\"},{\"content\":{\"connectorIds\":[\"Out1\"],\"side\":\"RIGHT\"},\"type\":\"ConnectorPlacement.EquallySpacedRectSide\",\"uuid\":\"a3669697-8e2e-4fce-83e7-11feb3c41a11\"},{\"content\":{\"connectorIds\":[\"In3\"],\"side\":\"TOP\"},\"type\":\"ConnectorPlacement.EquallySpacedRectSide\",\"uuid\":\"edbd7469-179d-4b36-ab80-dceaa86ef763\"},{\"content\":{\"side\":\"BOTTOM\"},\"type\":\"ConnectorPlacement.EquallySpacedRectSide\",\"uuid\":\"36ba3990-6628-4e3d-ab1a-10917dd4fa0b\"}]},\"type\":\"ConnectorPlacement.EquallySpacedConnector\",\"uuid\":\"68480e3c-12c2-4c1a-9580-60c15ea9a162\"}],\"packageUris\":[\"http://schema.mathworks.com/mf0/Connector/R2020b\"],\"version\":\"1.0\"}"
  Gain : Gain  Gain=params.capArea
  Gain2 : Gain  Gain=params.rodArea
  HECM : Subsystem
      settings: PortSchema="{\"entries\":[{\"content\":{\"sides\":[{\"content\":{\"connectorIds\":[\"In1\"]},\"type\":\"ConnectorPlacement.EquallySpacedRectSide\",\"uuid\":\"fa7e009b-3a28-4dd3-907b-76d8fd1f2fc5\"},{\"content\":{\"connectorIds\":[\"Out1\"],\"side\":\"RIGHT\"},\"type\":\"ConnectorPlacement.EquallySpacedRectSide\",\"uuid\":\"b4b71eb1-dc67-4897-9f20-563cedc71b8c\"},{\"content\":{\"connectorIds\":[\"In2\"],\"side\":\"TOP\"},\"type\":\"ConnectorPlacement.EquallySpacedRectSide\",\"uuid\":\"a67ddf4c-e1a7-4a41-beba-4c9482bc4896\"},{\"content\":{\"connectorIds\":[\"Out2\",\"In3\"],\"side\":\"BOTTOM\"},\"type\":\"ConnectorPlacement.EquallySpacedRectSide\",\"uuid\":\"d70e9d30-0c3d-4fe1-994c-11171af7a54f\"}]},\"type\":\"ConnectorPlacement.EquallySpacedConnector\",\"uuid\":\"d5f93414-5adb-4b46-aa3e-a0fd5f50c915\"}],\"packageUris\":[\"http://schema.mathworks.com/mf0/Connector/R2020b\"],\"version\":\"1.0\"}"
  Integrator : Integrator
  PressureRails : Subsystem
  Product : Product
  RodPressureDynamics : Subsystem
      settings: PortSchema="{\"entries\":[{\"content\":{\"sides\":[{\"content\":{\"connectorIds\":[\"In1\",\"In2\"]},\"type\":\"ConnectorPlacement.EquallySpacedRectSide\",\"uuid\":\"0a444e4d-7364-44e5-8b72-8c210fabafa0\"},{\"content\":{\"connectorIds\":[\"Out1\"],\"side\":\"RIGHT\"},\"type\":\"ConnectorPlacement.EquallySpacedRectSide\",\"uuid\":\"a3669697-8e2e-4fce-83e7-11feb3c41a11\"},{\"content\":{\"side\":\"TOP\"},\"type\":\"ConnectorPlacement.EquallySpacedRectSide\",\"uuid\":\"edbd7469-179d-4b36-ab80-dceaa86ef763\"},{\"content\":{\"connectorIds\":[\"In3\"],\"side\":\"BOTTOM\"},\"type\":\"ConnectorPlacement.EquallySpacedRectSide\",\"uuid\":\"0057cc85-602f-4ff7-8e06-c43254199496\"}]},\"type\":\"ConnectorPlacement.EquallySpacedConnector\",\"uuid\":\"68480e3c-12c2-4c1a-9580-60c15ea9a162\"}],\"packageUris\":[\"http://schema.mathworks.com/mf0/Connector/R2020b\"],\"version\":\"1.0\"}"
  Scope : Scope
  Scope1 : Scope  NumInputPorts=2
  To Workspace : ToWorkspace  VariableName=Energy  SampleTime=-1
      settings: MaxDataPoints=1
  capValves : Subsystem
      settings: PortSchema="{\"entries\":[{\"content\":{\"sides\":[{\"content\":{\"connectorIds\":[\"In1\",\"In2\"]},\"type\":\"ConnectorPlacement.EquallySpacedRectSide\",\"uuid\":\"d2e8cfa0-a0ae-49da-8fda-082dfd3b2d9f\"},{\"content\":{\"connectorIds\":[\"In3\"],\"side\":\"RIGHT\"},\"type\":\"ConnectorPlacement.EquallySpacedRectSide\",\"uuid\":\"7b83af61-76d6-4e35-9365-fafdba130762\"},{\"content\":{\"connectorIds\":[\"Out2\"],\"side\":\"TOP\"},\"type\":\"ConnectorPlacement.EquallySpacedRectSide\",\"uuid\":\"6880d985-ed9d-415d-a1a9-fc8aaf1ae9e0\"},{\"content\":{\"connectorIds\":[\"Out1\"],\"side\":\"BOTTOM\"},\"type\":\"ConnectorPlacement.EquallySpacedRectSide\",\"uuid\":\"f70b92c7-c6bf-4dbf-a331-364ba55ce8fb\"}]},\"type\":\"ConnectorPlacement.EquallySpacedConnector\",\"uuid\":\"7ffcaf2b-fb7f-4cb0-b739-43ebea45fc90\"}],\"packageUris\":[\"http://schema.mathworks.com/mf0/Connector/R2020b\"],\"version\":\"1.0\"}"
  rodValves : Subsystem
      settings: PortSchema="{\"entries\":[{\"content\":{\"sides\":[{\"content\":{\"connectorIds\":[\"In1\",\"In2\"]},\"type\":\"ConnectorPlacement.EquallySpacedRectSide\",\"uuid\":\"d2e8cfa0-a0ae-49da-8fda-082dfd3b2d9f\"},{\"content\":{\"connectorIds\":[\"In3\"],\"side\":\"RIGHT\"},\"type\":\"ConnectorPlacement.EquallySpacedRectSide\",\"uuid\":\"7b83af61-76d6-4e35-9365-fafdba130762\"},{\"content\":{\"connectorIds\":[\"Out2\"],\"side\":\"TOP\"},\"type\":\"ConnectorPlacement.EquallySpacedRectSide\",\"uuid\":\"6880d985-ed9d-415d-a1a9-fc8aaf1ae9e0\"},{\"content\":{\"connectorIds\":[\"Out1\"],\"side\":\"BOTTOM\"},\"type\":\"ConnectorPlacement.EquallySpacedRectSide\",\"uuid\":\"f70b92c7-c6bf-4dbf-a331-364ba55ce8fb\"}]},\"type\":\"ConnectorPlacement.EquallySpacedConnector\",\"uuid\":\"7ffcaf2b-fb7f-4cb0-b739-43ebea45fc90\"}],\"packageUris\":[\"http://schema.mathworks.com/mf0/Connector/R2020b\"],\"version\":\"1.0\"}"
  Force : Outport
  railPressure : Outport  Port=2
  capPressure : Outport  Port=3
  rodValvePressure : Outport  Port=4
  rodPressure : Outport  Port=5
  wires:
  Gain/1 -> Add/1
  RodPressureDynamics/1(rodPressure) -> Gain2/1, Scope1/2, rodPressure/1, HECM/3(rodPressure)  "rodPressure"
  rodValves/2(flow) -> HECM/1(flowIn)
  capValves/1(flow) -> CapPressureDynamics/3(flow)
  position/1 -> RodPressureDynamics/2(position), CapPressureDynamics/1(position)  "postion"
  Integrator/1 -> To Workspace/1, Scope/1  "Energy"
  velocity/1 -> Product/2, RodPressureDynamics/1(velocity), CapPressureDynamics/2(velocity)  "velocity"
  capValveCommands/1 -> capValves/2(valveCommands)
  CapPressureDynamics/1(capPressure) -> capPressure/1, capValves/3(Pout), Gain/1
  Product/1 -> Integrator/1  "Power"
  Add/1 -> Force/1, Product/1  "force"
  PressureRails/1(pressureRails) -> rodValves/2(railPressure), capValves/1(railPressure), railPressure/1
  rodValveCommands/1 -> rodValves/1(valveCommands)
  HECM/1(flowOut) -> RodPressureDynamics/3(flow)
  speedCommand/1 -> HECM/2(speedCommand)
  Gain2/1 -> Add/2
  HECM/2(rodValvePressure) -> rodValves/3(Pout), rodValvePressure/1
  "rodPressureCommand "/1 -> Scope1/1
  rodValves/1(railFlow) -> PressureRails/2(rodRailFlow)
  capValves/2(railFlow) -> PressureRails/1(capRailFlow)

== system Flap/PTO/Passive Valving/CapPressureDynamics ==
  position : Inport
  velocity : Inport  Port=2
  flow : Inport  Port=3
  Integrator : Integrator  LimitOutput=on  UpperSaturationLimit=30e6  LowerSaturationLimit=0
  MATLAB Function : MATLAB Function  TreatAsAtomicUnit=on
  capPressure : Outport
  wires:
  position/1 -> MATLAB Function/1(position)
  velocity/1 -> MATLAB Function/2(velocity)
  flow/1 -> MATLAB Function/3(flow)
  Integrator/1 -> capPressure/1  "capPressure"
  MATLAB Function/1(pressure_dot) -> Integrator/1  "capPressureDot"

== system Flap/PTO/Passive Valving/PressureRails ==
  note: flow into the rails
  capRailFlow : Inport
  rodRailFlow : Inport  Port=2
  Constant : Constant  Value=params.pressure
  Constant4 : Constant  Value=0
  Mux : Mux  Inputs=2
  Product : Product
  Sum : Sum  Inputs=|++
  Sum of Elements : Sum  Inputs=+
  To Workspace : ToWorkspace  VariableName=railPower  SampleTime=-1
  pressureRails : Outport
  wires:
  Mux/1 -> Product/2, pressureRails/1
  Constant4/1 -> Mux/1
  Constant/1 -> Mux/2
  Sum/1 -> Product/1
  Product/1 -> Sum of Elements/1
  Sum of Elements/1 -> To Workspace/1
  rodRailFlow/1 -> Sum/2
  capRailFlow/1 -> Sum/1

== system Flap/PTO/Passive Valving/RodPressureDynamics ==
  velocity : Inport
  position : Inport  Port=2
  flow : Inport  Port=3
  Integrator : Integrator  LimitOutput=on  UpperSaturationLimit=30e6  LowerSaturationLimit=0
  MATLAB Function : MATLAB Function  TreatAsAtomicUnit=on
  rodPressure : Outport
  wires:
  MATLAB Function/1(pressure_dot) -> Integrator/1
  Integrator/1 -> rodPressure/1  "rodPressure"
  flow/1 -> MATLAB Function/3(flow)
  velocity/1 -> MATLAB Function/2(velocity)
  position/1 -> MATLAB Function/1(position)

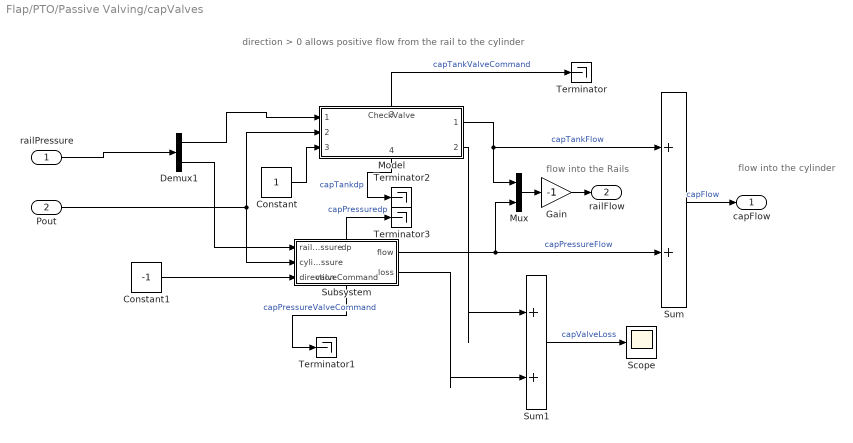
== system Flap/PTO/Passive Valving/capValves ==
  note: flow into the cylinder
  note: flow into the Rails
  note: direction > 0 allows positive flow from the rail to the cylinder
  railPressure : Inport
  Pout : Inport  Port=2
  Constant : Constant
  Constant1 : Constant  Value=-1
  Demux1 : Demux  Outputs=2
  Gain : Gain  Gain=-1
  Model : ModelReference  ModelNameDialog=CheckValve.slx  SimulationMode=Normal  ModelReferenceVersion=1.13
      settings: PortSchema="{\"entries\":[{\"content\":{\"sides\":[{\"content\":{\"connectorIds\":[\"In1\",\"In2\",\"In3\"]},\"type\":\"ConnectorPlacement.EquallySpacedRectSide\",\"uuid\":\"9926bc24-44a6-4299-a084-1660c4fff972\"},{\"content\":{\"connectorIds\":[\"Out1\",\"Out2\"],\"side\":\"RIGHT\"},\"type\":\"ConnectorPlacement.EquallySpacedRectSide\",\"uuid\":\"3da161dd-8b49-4c37-8c7c-74b1690709b5\"},{\"content\":{\"connectorIds\":[\"Out3\"],\"side\":\"TOP\"},\"type\":\"ConnectorPlacement.EquallySpacedRectSide\",\"uuid\":\"43f56c93-0008-49b1-aa20-7b8e5fa2b493\"},{\"content\":{\"connectorIds\":[\"Out4\"],\"side\":\"BOTTOM\"},\"type\":\"ConnectorPlacement.EquallySpacedRectSide\",\"uuid\":\"3d46221c-bbfd-47c3-8a33-074780286757\"}]},\"type\":\"ConnectorPlacement.EquallySpacedConnector\",\"uuid\":\"4c1266d4-f558-4b36-b773-481606d1abcf\"}],\"packageUris\":[\"http://schema.mathworks.com/mf0/Connector/R2020b\"],\"version\":\"1.0\"}"
  Mux : Mux  Inputs=2
  Scope : Scope
  Subsystem : Subsystem
      settings: PortSchema="{\"entries\":[{\"content\":{\"sides\":[{\"content\":{\"connectorIds\":[\"In1\",\"In2\",\"In3\"]},\"type\":\"ConnectorPlacement.EquallySpacedRectSide\",\"uuid\":\"18d55346-c99c-4c4a-9e28-cc9d0714d85d\"},{\"content\":{\"connectorIds\":[\"Out1\",\"Out2\"],\"side\":\"RIGHT\"},\"type\":\"ConnectorPlacement.EquallySpacedRectSide\",\"uuid\":\"f1e5d43e-01f0-4e52-b023-1f47868d6527\"},{\"content\":{\"connectorIds\":[\"Out4\"],\"side\":\"TOP\"},\"type\":\"ConnectorPlacement.EquallySpacedRectSide\",\"uuid\":\"ed947d41-aed1-4415-8729-4bc9599fec69\"},{\"content\":{\"connectorIds\":[\"Out3\"],\"side\":\"BOTTOM\"},\"type\":\"ConnectorPlacement.EquallySpacedRectSide\",\"uuid\":\"89145ef9-1aec-4fca-8a06-2cc22e7c3494\"}]},\"type\":\"ConnectorPlacement.EquallySpacedConnector\",\"uuid\":\"b1aebbf1-6707-46d0-a904-89d6e45951e7\"}],\"packageUris\":[\"http://schema.mathworks.com/mf0/Connector/R2020b\"],\"version\":\"1.0\"}"
  Sum : Sum
  Sum1 : Sum  Inputs=|++
  Terminator{,1..3} (4 alike) : Terminator
  capFlow : Outport
  railFlow : Outport  Port=2
  wires:
  Demux1/2 -> Subsystem/1(railPressure)
  Demux1/1 -> Model/1
  railPressure/1 -> Demux1/1
  Sum1/1 -> Scope/1  "capValveLoss"
  Subsystem/2(loss) -> Sum1/2
  Model/2 -> Sum1/1
  Sum/1 -> capFlow/1  "capFlow"
  Subsystem/1(flow) -> Mux/2, Sum/2  "capPressureFlow"
  Model/1 -> Mux/1, Sum/1  "capTankFlow"
  Constant1/1 -> Subsystem/3(direction)
  Pout/1 -> Subsystem/2(cylinderPressure), Model/2
  Mux/1 -> Gain/1
  Constant/1 -> Model/3
  Gain/1 -> railFlow/1
  Model/3 -> Terminator/1  "capTankValveCommand"
  Subsystem/3(valveCommand) -> Terminator1/1  "capPressureValveCommand"
  Model/4 -> Terminator2/1  "capTankdp"
  Subsystem/4(dp) -> Terminator3/1  "capPressuredp"

== system Flap/PTO/Passive Valving/rodValves ==
  note: direction > 0 allows positive flow from the rail to the cylinder
  note: flow into the cylinder
  note: flow into the Rails
  railPressure : Inport
  Pout : Inport  Port=2
  Constant : Constant
  Constant1 : Constant  Value=-1
  Demux1 : Demux  Outputs=2
  Gain : Gain  Gain=-1
  Model : ModelReference  ModelNameDialog=CheckValve.slx  SimulationMode=Normal  ModelReferenceVersion=1.13
  Model1 : ModelReference  ModelNameDialog=CheckValve.slx  SimulationMode=Normal  ModelReferenceVersion=1.13
  Mux : Mux  Inputs=2
  Scope : Scope
  Sum : Sum
  Sum1 : Sum  Inputs=|++
  railFlow : Outport
  rodFlow : Outport  Port=2
  wires:
  Demux1/1 -> Model/1
  railPressure/1 -> Demux1/1
  Sum1/1 -> Scope/1  "rodValveLoss"
  Model1/2 -> Sum1/2
  Model/2 -> Sum1/1
  Sum/1 -> rodFlow/1  "rodFlow"
  Constant1/1 -> Model1/3
  Demux1/2 -> Model1/1
  Constant/1 -> Model/3
  Pout/1 -> Model1/2, Model/2
  Model/1 -> Sum/1, Mux/1
  Model1/1 -> Mux/2, Sum/2
  Mux/1 -> Gain/1
  Gain/1 -> railFlow/1

== system Flap/PTO/Active Valving/capValves/Subsystem ==
  Pin : Inport
  Pout : Inport  Port=2
  valveCommand : Inport  Port=3
  MATLAB Function : MATLAB Function  TreatAsAtomicUnit=on
  flow : Outport
  loss : Outport  Port=2
  wires:
  MATLAB Function/1(flow) -> flow/1
  valveCommand/1 -> MATLAB Function/3(valveCommand)
  Pout/1 -> MATLAB Function/2(Pout)
  Pin/1 -> MATLAB Function/1(Pin)
  MATLAB Function/2(loss) -> loss/1
